simulink model "BrushlessMotorControlSim"  (R2021a)
settings: Solver=VariableStepAuto  StartTime=0.0  StopTime=tf  RelTol=1e-3
model workspace (MAT data in the model file):
  A = 1
values from neighbouring files (symbols this model uses):
  b = 0.5    [RunSimulation.m]
  D = 0    [RunSimulation.m]
  I = 4    [RunSimulation.m]
  J = 0.0002    [RunSimulation.m]
  Ke = 1.0    (= 1)    [RunSimulation.m]
  Kt = 1.0    (= 1)    [RunSimulation.m]
  L = 1    [RunSimulation.m]
  P = 1    [RunSimulation.m]
  R = 5    [RunSimulation.m]
  Ts = 0.10    (= 0.1)    [RunSimulation.m]
libraries: pid_lib x1
settings Model: Creator=alexj  LastModifiedBy=alexj

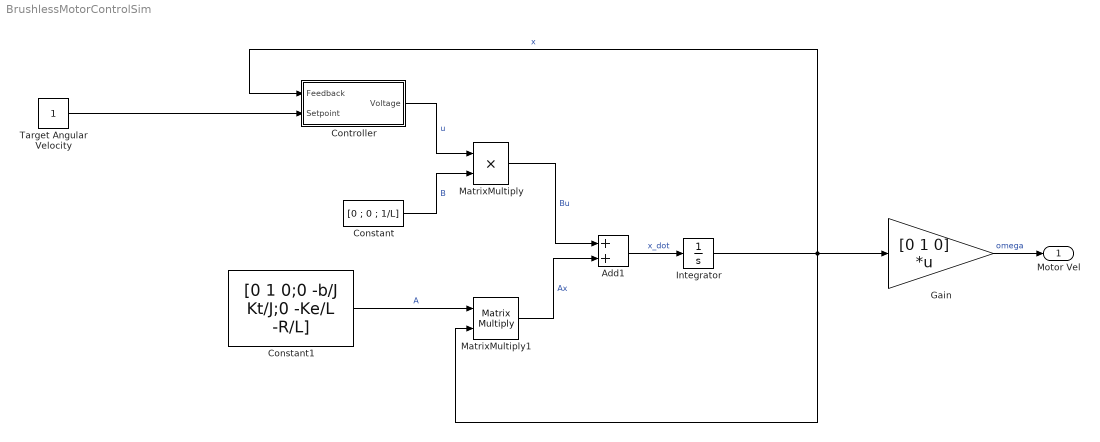
== system BrushlessMotorControlSim ==
  Add1 : Sum
  Constant : Constant  Value=[0 ; 0 ; 1/L]
  Constant1 : Constant  Value=[0 1 0;0 -b/J Kt/J;0 -Ke/L -R/L]
  Controller : Subsystem
  Gain : Gain  Gain=[0 1 0]  Multiplication=Matrix(K*u) (u vector)
  Integrator : Integrator  InitialCondition=[0;0;0]
  MatrixMultiply : Product
  MatrixMultiply1 : Product  Multiplication=Matrix(*)
  Target Angular Velocity : Constant
  Motor Vel : Outport
  wires:
  Controller/1(Voltage) -> MatrixMultiply/1  "u"
  Constant/1 -> MatrixMultiply/2  "B"
  MatrixMultiply/1 -> Add1/1  "Bu"
  Constant1/1 -> MatrixMultiply1/1  "A"
  MatrixMultiply1/1 -> Add1/2  "Ax"
  Add1/1 -> Integrator/1  "x_dot"
  Target Angular Velocity/1 -> Controller/2(Setpoint)
  Gain/1 -> Motor Vel/1  "omega"
  Integrator/1 -> Gain/1, Controller/1(Feedback), MatrixMultiply1/2  "x"

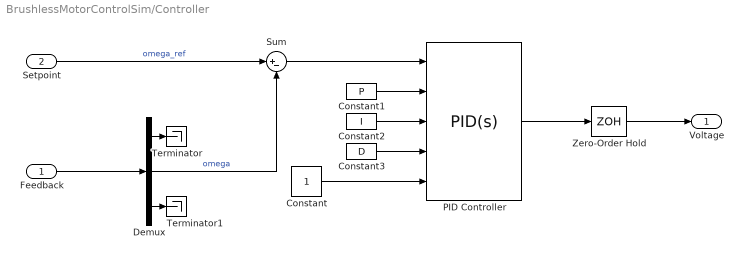
== system BrushlessMotorControlSim/Controller ==
  Feedback : Inport
  Setpoint : Inport  Port=2
  Constant : Constant
  Constant1 : Constant  Value=P
  Constant2 : Constant  Value=I
  Constant3 : Constant  Value=D
  Demux : Demux  Outputs=3
  PID Controller : pid_lib/PID Controller  Controller=PID  Form=Parallel  TimeDomain=Continuous-time  UseExternalTs=off  SampleTime=-1  IntegratorMethod=Forward Euler  FilterMethod=Forward Euler  ControllerParametersSource=external  P=1  I=1  D=0  UseFilter=on  N=100  TunerSelectOption=Transfer Function Based (PID Tuner App)  InitialConditionSource=internal  InitialConditionForIntegrator=0  InitialConditionForFilter=0  DifferentiatorICPrevScaledInput=0  ExternalReset=none  TrackingMode=off  Kt=1  LimitOutput=on  SatLimitsSource=internal  UpperSaturationLimit=12  LowerSaturationLimit=-12  LinearizeAsGain=off  AntiWindupMode=clamping  Kb=1  POutMin=[]  POutMax=[]  IOutMin=[]  IOutMax=[]  DOutMin=[]  DOutMax=[]  NOutMin=[]  NOutMax=[]  SumOutMin=[]  SumOutMax=[]  SaturationOutMin=[]  SaturationOutMax=[]  PParamMin=[]  PParamMax=[]  IParamMin=[]  IParamMax=[]  DParamMin=[]  DParamMax=[]  NParamMin=[]  NParamMax=[]  KbParamMin=[]  KbParamMax=[]  KtParamMin=[]  KtParamMax=[]  KbOutMin=[]  KbOutMax=[]  KtOutMin=[]  KtOutMax=[]  IntegratorOutMin=[]  IntegratorOutMax=[]  FilterOutMin=[]  FilterOutMax=[]  SumI1OutMin=[]  SumI1OutMax=[]  SumI2OutMin=[]  SumI2OutMax=[]  SumI3OutMin=[]  SumI3OutMax=[]  SumI4OutMin=[]  SumI4OutMax=[]  SumDOutMin=[]  SumDOutMax=[]  DifferentiatorOutMin=[]  DifferentiatorOutMax=[]  FilterDiffOutCoefMin=[]  FilterDiffOutCoefMax=[]  ReciprocalOutMin=[]  ReciprocalOutMax=[]  SumDenOutMin=[]  SumDenOutMax=[]  SumNumOutMin=[]  SumNumOutMax=[]  DivideOutMin=[]  DivideOutMax=[]  UdiffTsProdOutMin=[]  UdiffTsProdOutMax=[]  NTsProdOutMin=[]  NTsProdOutMax=[]  UintegralTsProdOutMin=[]  UintegralTsProdOutMax=[]  UngainTsProdOutMin=[]  UngainTsProdOutMax=[]  IntegratorContinuousStateAttributes=''  IntegratorStateMustResolveToSignalObject=off  IntegratorRTWStateStorageClass=Auto  FilterContinuousStateAttributes=''  FilterStateMustResolveToSignalObject=off  FilterRTWStateStorageClass=Auto  ParallelPVariant=ExternalParameters  IdealPVariant=Disabled  IVariant=ExternalParameters  DVariant=ExternalParameters  IntegratorVariant=Continuous  SatVariant=Enabled  AWVariant=ContClampingParallel  PCopyVariant=Disabled  TRVariant=Disabled  FdbkBlocksVariant=Forward  IdealPFdbkVariant=Disabled  SatFdbkVariant=Disabled  DerivativeFilterVariant=ContFilter  NVariant=ExternalParameters  NCopyVariant=Disabled  FilterICVariant=InternalICsFilter  IntegratorICVariant=InternalICs  ExternalResetVariant=Disabled  TRSumVariant=Passthrough  SumFdbkVariant=Disabled  SumVariant=Sum_PID  TsampFilterVariant=InternalTs  TsampNgainVariant=Passthrough  TsampIntegralVariant=Passthrough  ExternalSaturationOutDataTypeStr=Inherit: Same as second input
  Sum : Sum  Inputs=|+-
  Terminator : Terminator
  Terminator1 : Terminator
  Zero-Order Hold : ZeroOrderHold  SampleTime=Ts
  Voltage : Outport
  wires:
  Sum/1 -> PID Controller/1
  PID Controller/1 -> Zero-Order Hold/1
  Constant/1 -> PID Controller/5
  Constant1/1 -> PID Controller/2
  Constant2/1 -> PID Controller/3
  Constant3/1 -> PID Controller/4
  Demux/1 -> Terminator/1
  Demux/3 -> Terminator1/1
  Feedback/1 -> Demux/1
  Demux/2 -> Sum/2  "omega"
  Setpoint/1 -> Sum/1  "omega_ref"
  Zero-Order Hold/1 -> Voltage/1
